simulink model "Active_Suspension_PID_method_1"  (R2023a)
settings: Solver=VariableStepAuto  StartTime=0.0  StopTime=10  RelTol=1e-3
libraries: slpidlib x1
settings Model: Creator=CL606_24  LastModifiedBy=nanda
settings DebuggingCC: UnconnectedInputMsg=warning  UnconnectedOutputMsg=warning  UnconnectedLineMsg=warning
settings ModelReferenceCC: EnableRefExpFcnMdlSchedulingChecks=on
settings RTWCC: DLArmComputeVersion=19.05

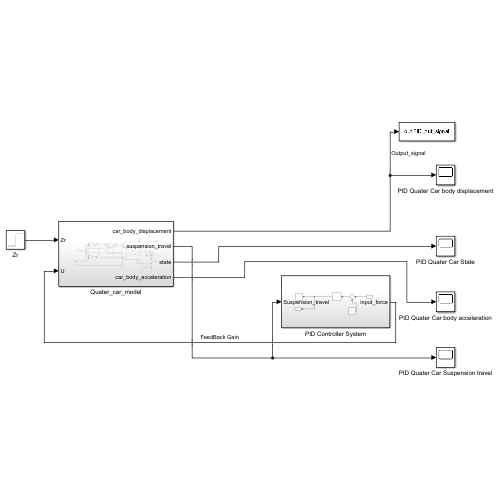
[thumbnail: Simulink's stored preview of the top-level diagram]
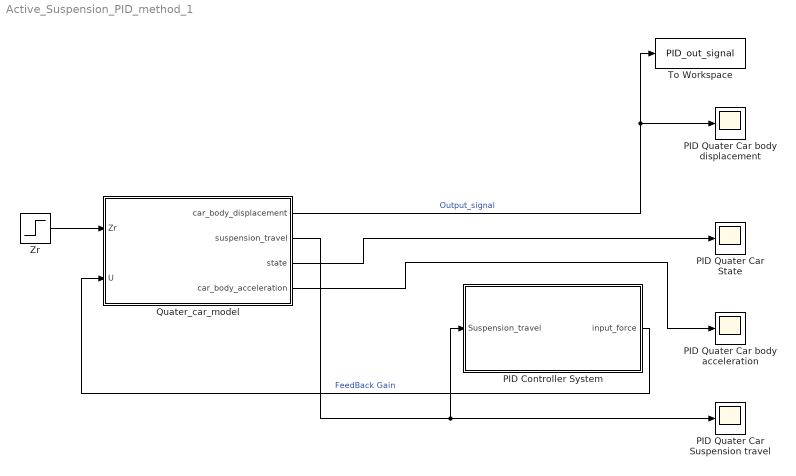
== system Active_Suspension_PID_method_1 ==
  PID Controller System : Subsystem
  PID Quater Car State : Scope
  PID Quater Car Suspension travel : Scope
  PID Quater Car body acceleration : Scope
  PID Quater Car body displacement : Scope
  Quater_car_model : Subsystem
  To Workspace : ToWorkspace  VariableName=PID_out_signal  SaveFormat=Structure With Time  SampleTime=-1
  Zr : Step  After=0.5  SampleTime=0
  wires:
  Zr/1 -> Quater_car_model/1(Zr)
  Quater_car_model/4(car_body_acceleration) -> PID Quater Car body acceleration/1
  Quater_car_model/1(car_body_displacement) -> To Workspace/1, PID Quater Car body displacement/1  "Output_signal"
  Quater_car_model/3(state) -> PID Quater Car State/1
  PID Controller System/1(input_force) -> Quater_car_model/2(U)  "FeedBack Gain"
  Quater_car_model/2(suspension_travel) -> PID Controller System/1(Suspension_travel), PID Quater Car Suspension travel/1

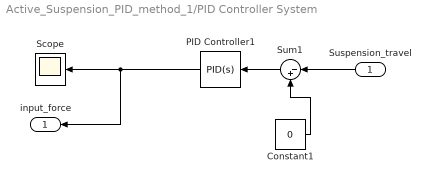
== system Active_Suspension_PID_method_1/PID Controller System ==
  Suspension_travel : Inport
  Constant1 : Constant  Value=0
  PID Controller1 : slpidlib/PID Controller  Controller=PID  Form=Parallel  TimeDomain=Continuous-time  UseExternalTs=off  SampleTime=-1  IntegratorMethod=Forward Euler  FilterMethod=Forward Euler  ControllerParametersSource=internal  P=-23856.0349273289  I=-60844.5106679341  UseKiTs=on  D=-2297.71257746443  N=1409.73193810167  UseFilter=on  TunerSelectOption=Transfer Function Based (PID Tuner App)  InitialConditionSource=internal  InitialConditionForIntegrator=0  InitialConditionForFilter=0  DifferentiatorICPrevScaledInput=0  ExternalReset=none  TrackingMode=off  Kt=1  LimitOutput=off  SatLimitsSource=internal  UpperSaturationLimit=inf  LowerSaturationLimit=-inf  LinearizeAsGain=on  AntiWindupMode=none  Kb=1  LimitIntegrator=off  UpperIntegratorSaturationLimit=inf  LowerIntegratorSaturationLimit=-inf  POutMin=[]  POutMax=[]  IOutMin=[]  IOutMax=[]  DOutMin=[]  DOutMax=[]  NOutMin=[]  NOutMax=[]  SumOutMin=[]  SumOutMax=[]  SaturationOutMin=[]  SaturationOutMax=[]  PParamMin=[]  PParamMax=[]  IParamMin=[]  IParamMax=[]  DParamMin=[]  DParamMax=[]  NParamMin=[]  NParamMax=[]  KbParamMin=[]  KbParamMax=[]  KtParamMin=[]  KtParamMax=[]  KbOutMin=[]  KbOutMax=[]  KtOutMin=[]  KtOutMax=[]  IntegratorOutMin=[]  IntegratorOutMax=[]  FilterOutMin=[]  FilterOutMax=[]  SumI1OutMin=[]  SumI1OutMax=[]  SumI2OutMin=[]  SumI2OutMax=[]  SumI3OutMin=[]  SumI3OutMax=[]  SumI4OutMin=[]  SumI4OutMax=[]  SumDOutMin=[]  SumDOutMax=[]  DifferentiatorOutMin=[]  DifferentiatorOutMax=[]  FilterDiffOutCoefMin=[]  FilterDiffOutCoefMax=[]  ReciprocalOutMin=[]  ReciprocalOutMax=[]  SumDenOutMin=[]  SumDenOutMax=[]  SumNumOutMin=[]  SumNumOutMax=[]  DivideOutMin=[]  DivideOutMax=[]  UdiffTsProdOutMin=[]  UdiffTsProdOutMax=[]  NTsProdOutMin=[]  NTsProdOutMax=[]  UintegralTsProdOutMin=[]  UintegralTsProdOutMax=[]  UngainTsProdOutMin=[]  UngainTsProdOutMax=[]  ClampingZeroOutDataTypeStr=Inherit: Inherit via back propagation  ClampingZeroOutMin=[]  ClampingZeroOutMax=[]  FilterDenConstantOutDataTypeStr=Inherit: Inherit via back propagation  FilterDenConstantOutMin=[]  FilterDenConstantOutMax=[]  PCopyOutDataTypeStr=Inherit: Inherit via back propagation  PCopyOutMin=[]  PCopyOutMax=[]  NCopyOutDataTypeStr=Inherit: Inherit via back propagation  NCopyOutMin=[]  NCopyOutMax=[]  IntegratorContinuousStateAttributes=''  IntegratorStateMustResolveToSignalObject=off  IntegratorRTWStateStorageClass=Auto  FilterContinuousStateAttributes=''  FilterStateMustResolveToSignalObject=off  FilterRTWStateStorageClass=Auto  ParallelPVariant=InternalParameters  IdealPVariant=Disabled  IVariant=InternalParameters  DVariant=InternalParameters  IntegratorVariant=Continuous  SatVariant=Disabled  AWVariant=Passthrough  PCopyVariant=Disabled  TRVariant=Disabled  FdbkBlocksVariant=Forward  IdealPFdbkVariant=Disabled  SatFdbkVariant=Disabled  DerivativeFilterVariant=ContFilter  NVariant=InternalParameters  NCopyVariant=Disabled  FilterICVariant=InternalICsFilter  IntegratorICVariant=InternalICs  ExternalResetVariant=Disabled  TRSumVariant=Passthrough  SumFdbkVariant=Disabled  SumVariant=Sum_PID  TsampFilterVariant=InternalTs  TsampNgainVariant=Passthrough  TsampIntegralVariant=Disabled_SignalSpec  ExternalSaturationOutDataTypeStr=Inherit: Same as second input
  Scope : Scope
  Sum1 : Sum  Inputs=|-+
  input_force : Outport
  wires:
  Suspension_travel/1 -> Sum1/1
  Sum1/1 -> PID Controller1/1
  Constant1/1 -> Sum1/2
  PID Controller1/1 -> input_force/1, Scope/1

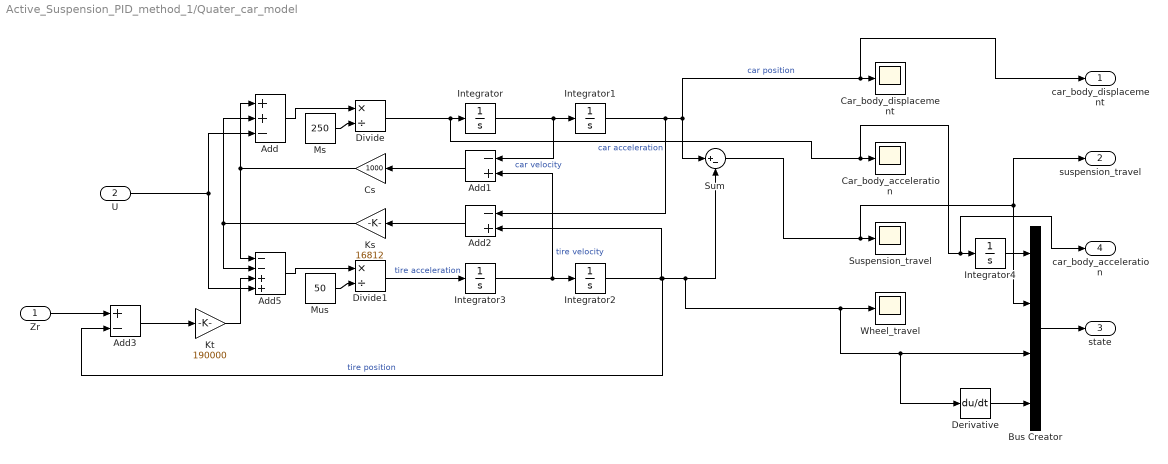
== system Active_Suspension_PID_method_1/Quater_car_model ==
  Zr : Inport
  U : Inport  Port=2
  Add : Sum  Inputs=++-
  Add1 : Sum  Inputs=-+
  Add2 : Sum  Inputs=-+
  Add3 : Sum  Inputs=+-
  Add5 : Sum  Inputs=--++
  Bus Creator : BusCreator  Inputs=4
  Car_body_acceleration : Scope
  Car_body_displacement : Scope
  Cs : Gain  Gain=1000
  Derivative : Derivative
  Divide : Product  Inputs=*/
  Divide1 : Product  Inputs=*/
  Integrator{,1..4} (5 alike) : Integrator
  Ks : Gain  Gain=16812
  Kt : Gain  Gain=190000
  Ms : Constant  Value=250
  Mus : Constant  Value=50
  Sum : Sum  Inputs=|+-
  Suspension_travel : Scope
  Wheel_travel : Scope
  car_body_displacement : Outport
  suspension_travel : Outport  Port=2
  state : Outport  Port=3
  car_body_acceleration : Outport  Port=4
  wires:
  Derivative/1 -> Bus Creator/4
  Integrator4/1 -> Bus Creator/1
  Integrator1/1 -> car_body_displacement/1, Car_body_displacement/1, Sum/1, Add2/1  "car position"
  Add1/1 -> Cs/1
  Divide1/1 -> Integrator3/1  "tire acceleration"
  Mus/1 -> Divide1/2
  Integrator3/1 -> Integrator2/1, Add1/2  "tire velocity"
  Sum/1 -> suspension_travel/1, Bus Creator/2, Suspension_travel/1
  Cs/1 -> Add/1, Add5/1
  Divide/1 -> car_body_acceleration/1, Integrator4/1, Car_body_acceleration/1, Integrator/1  "car acceleration"
  Kt/1 -> Add5/3
  Integrator2/1 -> Add3/2, Wheel_travel/1, Derivative/1, Bus Creator/3, Sum/2, Add2/2  "tire position"
  Integrator/1 -> Integrator1/1, Add1/1  "car velocity"
  Ks/1 -> Add5/2, Add/2
  Add2/1 -> Ks/1
  Add5/1 -> Divide1/1
  Add/1 -> Divide/1
  Ms/1 -> Divide/2
  Bus Creator/1 -> state/1
  U/1 -> Add/3, Add5/4
  Add3/1 -> Kt/1
  Zr/1 -> Add3/1
